simulink model "project1"  (R2020b)
settings: Solver=VariableStepAuto  StartTime=0.0  StopTime=10.0  RelTol=1e-3
undefined symbols (not defined in the file): b, k1, M1
settings Model: Creator=RASIKA MALGI  LastModifiedBy=RASIKA MALGI

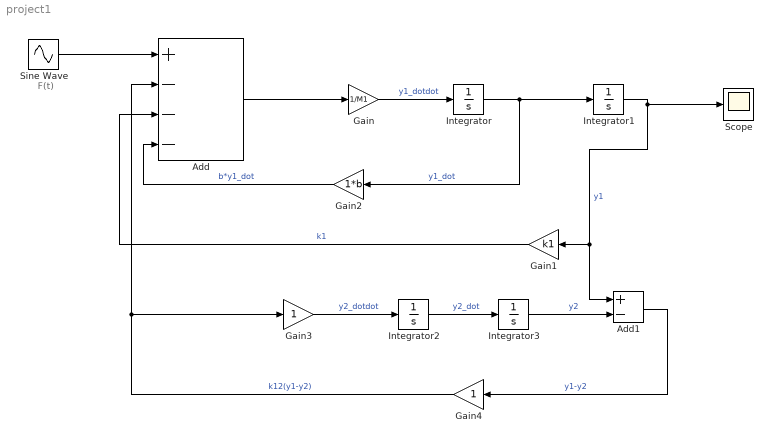
== system project1 ==
  note: F(t)
  Add : Sum  Inputs=+---
  Add1 : Sum  Inputs=+-
  Gain : Gain  Gain=1/M1
  Gain1 : Gain  Gain=k1
  Gain2 : Gain  Gain=1*b
  Gain3 : Gain
  Gain4 : Gain
  Integrator{,1..3} (4 alike) : Integrator
  Scope : Scope
  Sine Wave : Sin  SampleTime=0
  wires:
  Add/1 -> Gain/1
  Gain/1 -> Integrator/1  "y1_dotdot"
  Integrator/1 -> Gain2/1, Integrator1/1  "y1_dot"
  Sine Wave/1 -> Add/1
  Integrator1/1 -> Scope/1, Gain1/1, Add1/1  "y1"
  Integrator3/1 -> Add1/2  "y2"
  Integrator2/1 -> Integrator3/1  "y2_dot"
  Gain3/1 -> Integrator2/1  "y2_dotdot"
  Add1/1 -> Gain4/1  "y1-y2"
  Gain2/1 -> Add/4  "b*y1_dot"
  Gain1/1 -> Add/3  "k1"
  Gain4/1 -> Gain3/1, Add/2  "k12(y1-y2)"
